simulink model "Problem_3"  (R2020a)
settings: Solver=VariableStepAuto  StartTime=0.0  StopTime=100  RelTol=1e-3
PreLoadFcn:
  | m = 1000;
  | b = 50;
  | u = 500;
settings Model: DataDictionary=Dictionary_Problem3.sldd  Creator=Admin  LastModifiedBy=Admin

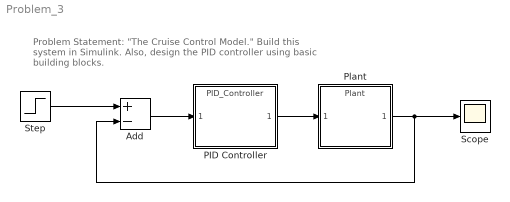
== system Problem_3 ==
  note: Problem Statement:
      | "The Cruise Control Model." Build this system in Simulink.
      | Also, design the PID controller using basic building blocks.
  Add : Sum  Inputs=+-
  PID Controller : ModelReference  ModelNameDialog=PID_Controller  ModelReferenceVersion=1.19
  Plant : ModelReference  ModelNameDialog=Plant  ModelReferenceVersion=1.18
  Scope : Scope
  Step : Step  Time=0  After=500  SampleTime=0
  wires:
  Plant/1 -> Add/2, Scope/1
  Step/1 -> Add/1
  Add/1 -> PID Controller/1
  PID Controller/1 -> Plant/1
